simulink library "simlib"  (R2019b)
settings: Solver=VariableStepAuto  StartTime=0.0  StopTime=10.0  RelTol=1e-3
settings Model: Creator=MusA  LastModifiedBy=MusA

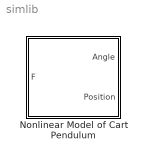
== system simlib ==
  Nonlinear Model of Cart Pendulum : Subsystem  mask{bf=0.1, cm=0.5, pm=0.2, l=0.3, g=9.81}
      mask prompts: bf "Cart Frac (N/m)"; cm "Cart Mass (kg)"; pm "pendu mass"; l "pendulum length"; g "gravit"
      mask Display: image('C:\Users\MusA\Documents\MATLAB\control\img\cartPendulum.png'); % Use "Edit Image" on toolstrip to change.

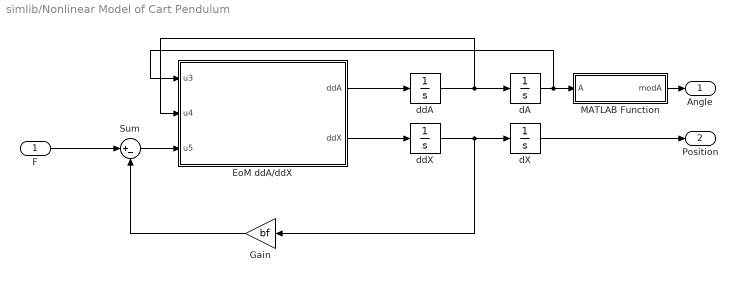
== system simlib/Nonlinear Model of Cart Pendulum ==
  F : Inport
  EoM ddA/ddX : MATLAB Function  TreatAsAtomicUnit=on
  Gain : Gain  Gain=bf
  MATLAB Function : MATLAB Function  TreatAsAtomicUnit=on
  Sum : Sum  Inputs=|+-
  dA : Integrator
  dX : Integrator
  ddA : Integrator
  ddX : Integrator
  Angle : Outport
  Position : Outport  Port=2
  wires:
  dA/1 -> EoM ddA/ddX/1(u3), MATLAB Function/1(A)
  EoM ddA/ddX/1(ddA) -> ddA/1
  ddA/1 -> EoM ddA/ddX/2(u4), dA/1
  ddX/1 -> Gain/1, dX/1
  Sum/1 -> EoM ddA/ddX/3(u5)
  EoM ddA/ddX/2(ddX) -> ddX/1
  MATLAB Function/1(modA) -> Angle/1
  dX/1 -> Position/1
  F/1 -> Sum/1
  Gain/1 -> Sum/2

== matlab function simlib/Nonlinear Model of Cart Pendulum/MATLAB Function ==
  data: A input; modA output
function modA = fcn(A)

% DESCRIPTION :
%         mod(A,2pi)between -pi/pi
%  Input:
%        A: alpha pendulum angle (radian)
%  Output:
%        modA: mod of Angle 
%  Required Functions : -
%  
%  NOTES :
%       Tags: #control #pendulum #mod #equation 
%       Copyright: licensed under Apache 2.0
% 
%  Date     Changes         Name                                                      
%  25May20  Created         Mus A (https://github.com/musa)

%%
A=A+pi;
positiveInput = (A > 0);
modA = mod(A, 2*pi);
modA((modA == 0) & positiveInput) = 2*pi;
modA=modA-pi;

== matlab function simlib/Nonlinear Model of Cart Pendulum/EoM ddA//ddX ==
  data: u3 input; ddA output; u4 input; u5 input; ddX output; g parameter; cm parameter; pm parameter; l parameter
function [ddA,ddX] = fcn(u3,u4,u5, g, cm, pm, l)

% DESCRIPTION :
%         Lagrangian equation of motion cart-pendulum
%  Input:
%        u3: alpha pendulum angle (radian)
%        u4: angular velocity of pendulum angle (radian/s)
%        u5: Cart total forces (F-bx) N
%        g: parameter - gravitational constant 9.81 kgm/s^2
%        cm: parameter - cart mass kg
%        pm: parameter - pendulum point mass kg
%        l: parameter - pendulum length cart to pendulum cog m
%  Output:
%        ddA: Angular accelaration radian/s^2
%        ddX: Horizantal cart position accelaration m/s^2
%  Required Functions : Change constant parameters
%  
%  NOTES :
%       Tags: #control #pendulum #model #equation
%       Copyright: licensed under Apache 2.0
% 
%  Date     Changes         Name                                                      
%  25May20  Created         Mus A (https://github.com/musa)

%%
ddX =(u5+pm*sin(u3)*(l*u4^2-g*cos(u3)))/(cm+pm*sin(u3)^2);
ddA=(-u5*cos(u3)-pm*l*u4^2*sin(u3)*cos(u3)+(cm+pm)*g*sin(u3))/(l*(cm+pm*sin(u3)^2));
